simulink model "hw2_0825_simulink"  (R2024a)
settings: Solver=VariableStepAuto  StartTime=0.0  StopTime=10.0  RelTol=1e-3
settings Model: Creator=karen  LastModifiedBy=karen

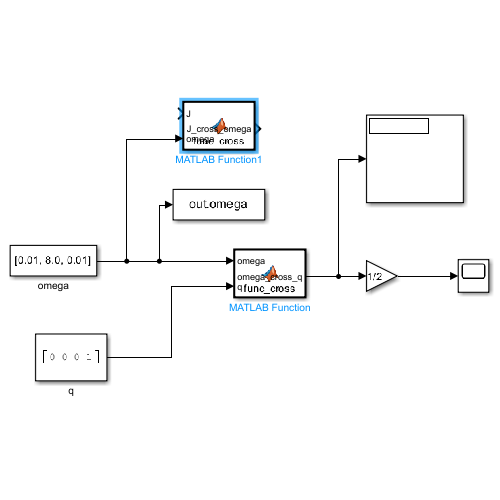
[thumbnail: Simulink's stored preview of the top-level diagram]
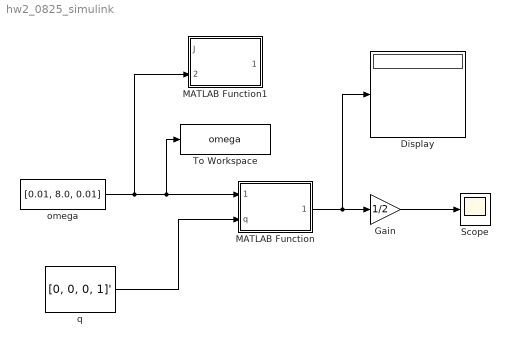
== system hw2_0825_simulink ==
  Display : Display
  Gain : Gain  Gain=1/2
  MATLAB Function : MATLAB Function  TreatAsAtomicUnit=on
  MATLAB Function1 : MATLAB Function  TreatAsAtomicUnit=on
  Scope : Scope
  To Workspace : ToWorkspace  VariableName=omega  SaveFormat=Timeseries  SampleTime=-1
  omega : Constant  Value=[0.01, 8.0, 0.01]
  q : Constant  Value=[0, 0, 0, 1]'
  wires:
  omega/1 -> MATLAB Function1/2(omega), To Workspace/1, MATLAB Function/1(omega)
  MATLAB Function/1(omega_cross_q) -> Display/1, Gain/1
  Gain/1 -> Scope/1
  q/1 -> MATLAB Function/2(q)

== matlab function hw2_0825_simulink/MATLAB Function ==
  data: omega input; omega_cross_q output; q input
function omega_cross_q = func_cross(omega,q)
  Omega = [0, omega(3), -omega(2) omega(1);
           -omega(3), 0, omega(1) omega(2);
           omega(2), -omega(1), 0, omega(3);
           -omega(1), -omega(2), -omega(3), 0];

  omega_cross_q = Omega * q;

end

== matlab function hw2_0825_simulink/MATLAB Function1 ==
  data: J input; J_cross_omega output; omega input
function J_cross_omega = func_cross(J,omega)
  
  J = [Ixx, 0, 0;
       0, Iyy, 0;
       0, 0, Izz];

  J_cross_omega = J * omega;

end
